simulink model "Neurofeedback_Full_fNIRS"  (R2021b)
settings: Solver=ode23tb  StartTime=0  StopTime=90  FixedStep=1/100  RelTol=1e-3
libraries: slpidlib x1
settings Model: Creator=mdls3  LastModifiedBy=mdls3
settings DataIOCC: SaveFormat=StructureWithTime
settings OptimizationCC: BlockReduction=off  BufferReuse=off
settings DebuggingCC: AlgebraicLoopMsg=none  UnconnectedInputMsg=none  UnconnectedOutputMsg=none  UnconnectedLineMsg=none  UnderSpecifiedDimensionMsg=warning

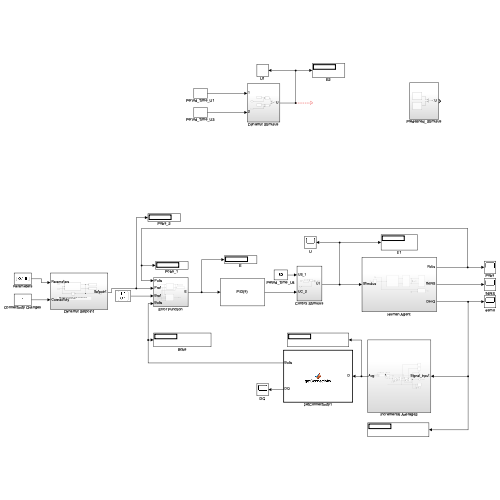
[thumbnail: Simulink's stored preview of the top-level diagram]
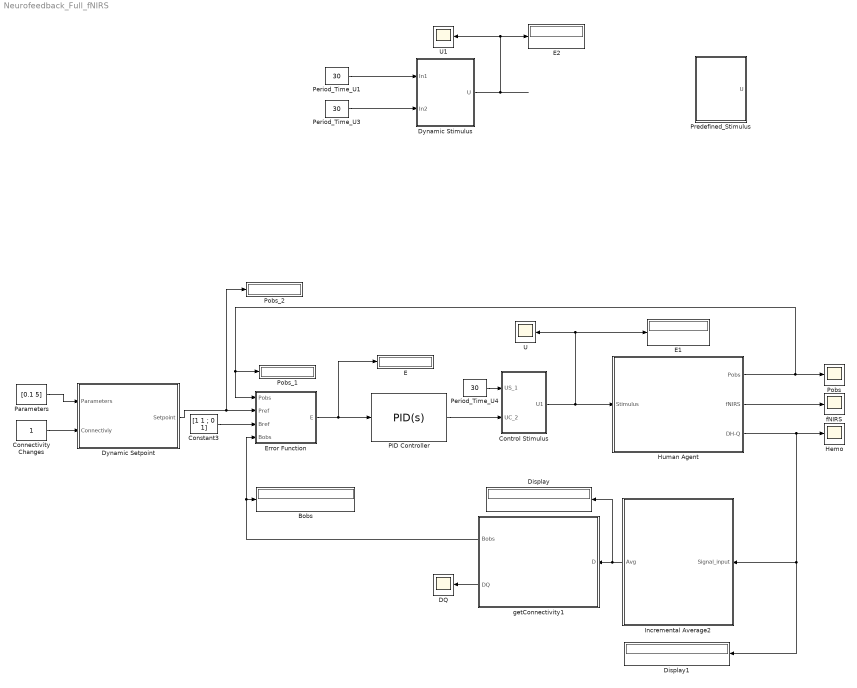
== system Neurofeedback_Full_fNIRS ==
  Bobs : Display
  Connectivity Changes : Constant
  Constant3 : Constant  Value="[1   1 ; 0  1]"
  Control Stimulus : Subsystem
  DQ : Scope
  Display : Display
  Display1 : Display
  Dynamic Setpoint : Subsystem
  Dynamic Stimulus : Subsystem
  E : Display
  E1 : Display
  E2 : Display
  Error Function : Subsystem
  Hemo : Scope
  Human Agent : Subsystem
  Incremental Average2 : Subsystem
  PID Controller : slpidlib/PID Controller  Controller=PID  Form=Ideal  TimeDomain=Continuous-time  UseExternalTs=off  SampleTime=-1  IntegratorMethod=Forward Euler  FilterMethod=Forward Euler  ControllerParametersSource=internal  P=0.3  I=0.12  D=0.85  UseFilter=on  N=100  TunerSelectOption=Transfer Function Based (PID Tuner App)  InitialConditionSource=internal  InitialConditionForIntegrator=0  InitialConditionForFilter=0  DifferentiatorICPrevScaledInput=0  ExternalReset=none  TrackingMode=off  Kt=1  LimitOutput=off  SatLimitsSource=internal  UpperSaturationLimit=inf  LowerSaturationLimit=-inf  LinearizeAsGain=on  AntiWindupMode=none  Kb=1  POutMin=[]  POutMax=[]  IOutMin=[]  IOutMax=[]  DOutMin=[]  DOutMax=[]  NOutMin=[]  NOutMax=[]  SumOutMin=[]  SumOutMax=[]  SaturationOutMin=[]  SaturationOutMax=[]  PParamMin=[]  PParamMax=[]  IParamMin=[]  IParamMax=[]  DParamMin=[]  DParamMax=[]  NParamMin=[]  NParamMax=[]  KbParamMin=[]  KbParamMax=[]  KtParamMin=[]  KtParamMax=[]  KbOutMin=[]  KbOutMax=[]  KtOutMin=[]  KtOutMax=[]  IntegratorOutMin=[]  IntegratorOutMax=[]  FilterOutMin=[]  FilterOutMax=[]  SumI1OutMin=[]  SumI1OutMax=[]  SumI2OutMin=[]  SumI2OutMax=[]  SumI3OutMin=[]  SumI3OutMax=[]  SumI4OutMin=[]  SumI4OutMax=[]  SumDOutMin=[]  SumDOutMax=[]  DifferentiatorOutMin=[]  DifferentiatorOutMax=[]  FilterDiffOutCoefMin=[]  FilterDiffOutCoefMax=[]  ReciprocalOutMin=[]  ReciprocalOutMax=[]  SumDenOutMin=[]  SumDenOutMax=[]  SumNumOutMin=[]  SumNumOutMax=[]  DivideOutMin=[]  DivideOutMax=[]  UdiffTsProdOutMin=[]  UdiffTsProdOutMax=[]  NTsProdOutMin=[]  NTsProdOutMax=[]  UintegralTsProdOutMin=[]  UintegralTsProdOutMax=[]  UngainTsProdOutMin=[]  UngainTsProdOutMax=[]  IntegratorContinuousStateAttributes=''  IntegratorStateMustResolveToSignalObject=off  IntegratorRTWStateStorageClass=Auto  FilterContinuousStateAttributes=''  FilterStateMustResolveToSignalObject=off  FilterRTWStateStorageClass=Auto  ParallelPVariant=Passthrough  IdealPVariant=InternalParameters  IVariant=InternalParameters  DVariant=InternalParameters  IntegratorVariant=Continuous  SatVariant=Disabled  AWVariant=Passthrough  PCopyVariant=Disabled  TRVariant=Disabled  FdbkBlocksVariant=Forward  IdealPFdbkVariant=Disabled  SatFdbkVariant=Disabled  DerivativeFilterVariant=ContFilter  NVariant=InternalParameters  NCopyVariant=Disabled  FilterICVariant=InternalICsFilter  IntegratorICVariant=InternalICs  ExternalResetVariant=Disabled  TRSumVariant=Passthrough  SumFdbkVariant=Disabled  SumVariant=Sum_PID  TsampFilterVariant=InternalTs  TsampNgainVariant=Passthrough  TsampIntegralVariant=Passthrough  ExternalSaturationOutDataTypeStr=Inherit: Same as second input
  Parameters : Constant  Value=[0.1 5]
  Period_Time_U1 : Constant  Value=30
  Period_Time_U3 : Constant  Value=30
  Period_Time_U4 : Constant  Value=30
  Pobs : Scope
  Pobs_1 : Display
  Pobs_2 : Display
  Predefined_Stimulus : Subsystem
  U : Scope
  U1 : Scope
  fNIRS : Scope
  getConnectivity1 : MATLAB Function  TreatAsAtomicUnit=on  SystemSampleTime=0
  wires:
  Constant3/1 -> Error Function/3(Bref)
  Dynamic Setpoint/1(Setpoint) -> Pobs_2/1, Error Function/2(Pref)
  Error Function/1(E) -> PID Controller/1, E/1
  Period_Time_U4/1 -> Control Stimulus/1(US_1)
  Period_Time_U1/1 -> Dynamic Stimulus/1(In1)
  Period_Time_U3/1 -> Dynamic Stimulus/2(In2)
  Dynamic Stimulus/1(U) -> E2/1, U1/1
  PID Controller/1 -> Control Stimulus/2(UC_2)
  Human Agent/1(Pobs) -> Pobs/1, Pobs_1/1, Error Function/1(Pobs)
  Human Agent/2(fNIRS) -> fNIRS/1
  Control Stimulus/1(U1) -> U/1, E1/1, Human Agent/1(Stimulus)
  Human Agent/3(DH-Q) -> Display1/1, Incremental Average2/1(Signal_input), Hemo/1
  Incremental Average2/1(Avg) -> Display/1, getConnectivity1/1("D ")
  getConnectivity1/2(DQ) -> DQ/1
  getConnectivity1/1(Bobs) -> Error Function/4(Bobs), Bobs/1
  Parameters/1 -> Dynamic Setpoint/1(Parameters)
  Connectivity Changes/1 -> Dynamic Setpoint/2(Connectiviy)

== system Neurofeedback_Full_fNIRS/Control Stimulus ==
  US_1 : Inport
  UC_2 : Inport  Port=2
  Duty_Cycle_U1 : Constant  Value=0.16667  OutMin=[0]  OutMax=[0.8]
  Mux : Mux  Inputs=2
  Variable Pulse Generator2 : VariablePulseGenerator  RunAtFixedTimeIntervals=on  SampleTime=1/100
  U1 : Outport
  wires:
  Duty_Cycle_U1/1 -> Variable Pulse Generator2/1
  US_1/1 -> Variable Pulse Generator2/2
  Variable Pulse Generator2/1 -> Mux/1
  UC_2/1 -> Mux/2
  Mux/1 -> U1/1

== system Neurofeedback_Full_fNIRS/Dynamic Setpoint ==
  note: It’s necessary to delete the random term and move it to change its connectivity changes.
  Parameters : Inport
  Connectiviy : Inport  Port=2
  Delay1 : Delay  DelayLength=1  InitialCondition=0
  MATLAB Function1 : MATLAB Function  TreatAsAtomicUnit=on
  Random : Display
  Set1 : Display
  Setpoint : Outport
  wires:
  Parameters/1 -> MATLAB Function1/1(Parameters)
  MATLAB Function1/2(random) -> Random/1
  MATLAB Function1/1(Setpoint) -> Set1/1, Setpoint/1, Delay1/1
  Delay1/1 -> MATLAB Function1/2(Last_pressure)
  Connectiviy/1 -> MATLAB Function1/3(Connectivity)

== system Neurofeedback_Full_fNIRS/Dynamic Stimulus ==
  In1 : Inport
  In2 : Inport  Port=2
  Duty_Cycle_U1 : Constant  Value=0.16667  OutMin=[0]  OutMax=[0.8]
  Duty_Cycle_U2 : Constant  Value=0.5  OutMin=[0]  OutMax=[0.8]
  Mux : Mux  Inputs=2
  Variable Pulse Generator1 : VariablePulseGenerator  RunAtFixedTimeIntervals=on  SampleTime=1/100
  Variable Pulse Generator2 : VariablePulseGenerator  RunAtFixedTimeIntervals=on  SampleTime=1/100
  U : Outport
  wires:
  In1/1 -> Variable Pulse Generator2/2
  Mux/1 -> U/1
  Variable Pulse Generator2/1 -> Mux/1
  Duty_Cycle_U1/1 -> Variable Pulse Generator2/1
  Duty_Cycle_U2/1 -> Variable Pulse Generator1/1
  In2/1 -> Variable Pulse Generator1/2
  Variable Pulse Generator1/1 -> Mux/2

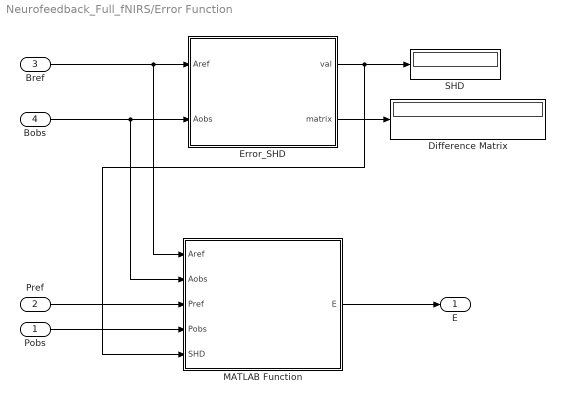
== system Neurofeedback_Full_fNIRS/Error Function ==
  Pobs : Inport
  Pref : Inport  Port=2
  Bref : Inport  Port=3
  Bobs : Inport  Port=4
  Difference Matrix : Display
  Error_SHD : MATLAB Function  TreatAsAtomicUnit=on
  MATLAB Function : MATLAB Function  TreatAsAtomicUnit=on
  SHD : Display
  E : Outport
  wires:
  Error_SHD/2(matrix) -> Difference Matrix/1
  Bref/1 -> MATLAB Function/1(Aref), Error_SHD/1(Aref)
  Error_SHD/1(val) -> SHD/1, MATLAB Function/5(SHD)
  MATLAB Function/1(E) -> E/1
  Bobs/1 -> MATLAB Function/2(Aobs), Error_SHD/2(Aobs)
  Pobs/1 -> MATLAB Function/4(Pobs)
  Pref/1 -> MATLAB Function/3(Pref)

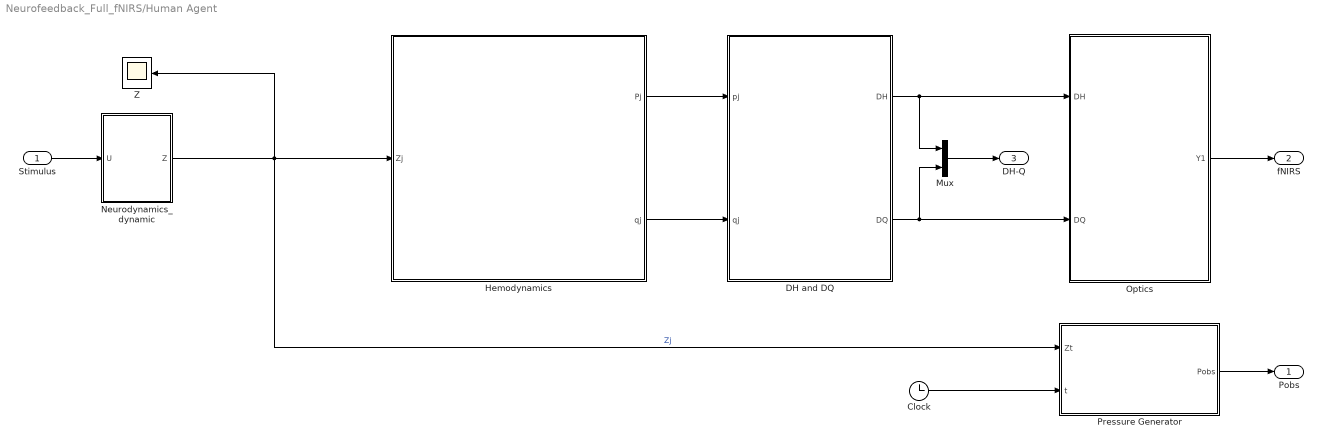
== system Neurofeedback_Full_fNIRS/Human Agent ==
  Stimulus : Inport
  Clock : Clock
  DH and DQ : Subsystem
  Hemodynamics : Subsystem
  Mux : Mux  Inputs=2
  Neurodynamics_dynamic : Subsystem
  Optics : Subsystem
  Pressure Generator : MATLAB Function  TreatAsAtomicUnit=on
  Z : Scope
  Pobs : Outport
  fNIRS : Outport  Port=2
  DH-Q : Outport  Port=3
  wires:
  Hemodynamics/1(Pj) -> DH and DQ/1(pj)
  Hemodynamics/2(qj) -> DH and DQ/2(qj)
  Neurodynamics_dynamic/1(Z) -> Hemodynamics/1(Zj), Z/1, Pressure Generator/1(Zt)  "Zj"
  DH and DQ/2(DQ) -> Mux/2, Optics/2(DQ)
  Optics/1(Y1) -> fNIRS/1
  Clock/1 -> Pressure Generator/2(t)
  Pressure Generator/1(Pobs) -> Pobs/1
  Stimulus/1 -> Neurodynamics_dynamic/1(U)
  DH and DQ/1(DH) -> Mux/1, Optics/1(DH)
  Mux/1 -> DH-Q/1

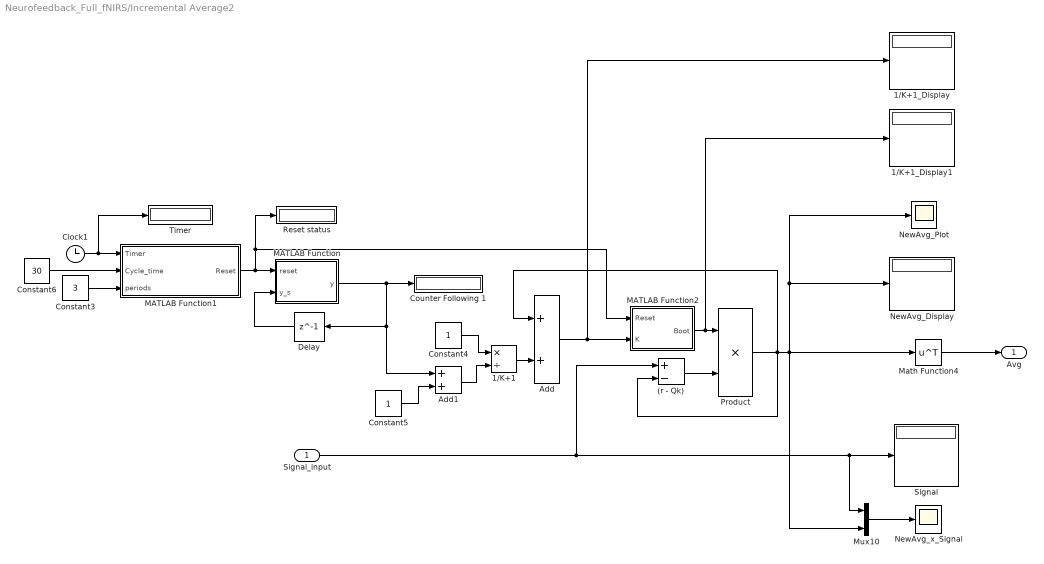
== system Neurofeedback_Full_fNIRS/Incremental Average2 ==
  Signal_input : Inport
  (r - Qk) : Sum  Inputs=+-
  1/K+1 : Product  Inputs=*/
  1/K+1_Display : Display
  1/K+1_Display1 : Display
  Add : Sum
  Add1 : Sum
  Clock1 : Clock
  Constant3 : Constant  Value=3
  Constant4 : Constant
  Constant5 : Constant
  Constant6 : Constant  Value=30
  Counter Following 1 : Display
  Delay : Delay  DelayLength=1  InitialCondition=0
  MATLAB Function : MATLAB Function  TreatAsAtomicUnit=on
  MATLAB Function1 : MATLAB Function  TreatAsAtomicUnit=on
  MATLAB Function2 : MATLAB Function  TreatAsAtomicUnit=on
  Math Function4 : Math  Operator=transpose  SaturateOnIntegerOverflow=on
  Mux10 : Mux  Inputs=2
  NewAvg_Display : Display
  NewAvg_Plot : Scope
  NewAvg_x_Signal : Scope
  Product : Product
  Reset status : Display
  Signal : Display
  Timer : Display
  Avg : Outport
  wires:
  (r - Qk)/1 -> Product/2
  Signal_input/1 -> Mux10/1, Signal/1, (r - Qk)/1
  Add/1 -> 1/K+1_Display/1, MATLAB Function2/2(K)
  Mux10/1 -> NewAvg_x_Signal/1
  Product/1 -> Add/1, (r - Qk)/2, Mux10/2, NewAvg_Plot/1, NewAvg_Display/1, Math Function4/1
  Math Function4/1 -> Avg/1
  Constant4/1 -> 1/K+1/1
  Constant5/1 -> Add1/2
  Add1/1 -> 1/K+1/2
  1/K+1/1 -> Add/2
  MATLAB Function/1(y) -> Delay/1, Add1/1, Counter Following 1/1
  Delay/1 -> MATLAB Function/2(y_s)
  MATLAB Function1/1(Reset) -> Reset status/1, MATLAB Function2/1(Reset), MATLAB Function/1(reset)
  Constant6/1 -> MATLAB Function1/2(Cycle_time)
  Constant3/1 -> MATLAB Function1/3(periods)
  Clock1/1 -> MATLAB Function1/1(Timer), Timer/1
  MATLAB Function2/1(Boot) -> 1/K+1_Display1/1, Product/1

== system Neurofeedback_Full_fNIRS/Predefined_Stimulus ==
  Mux : Mux  Inputs=2
  Pulse Generator : DiscretePulseGenerator  Amplitude=0.6  Period=30  PulseWidth=5
  Pulse Generator1 : DiscretePulseGenerator  Amplitude=0.6  Period=30  PulseWidth=6
  U : Outport
  wires:
  Mux/1 -> U/1
  Pulse Generator/1 -> Mux/1
  Pulse Generator1/1 -> Mux/2

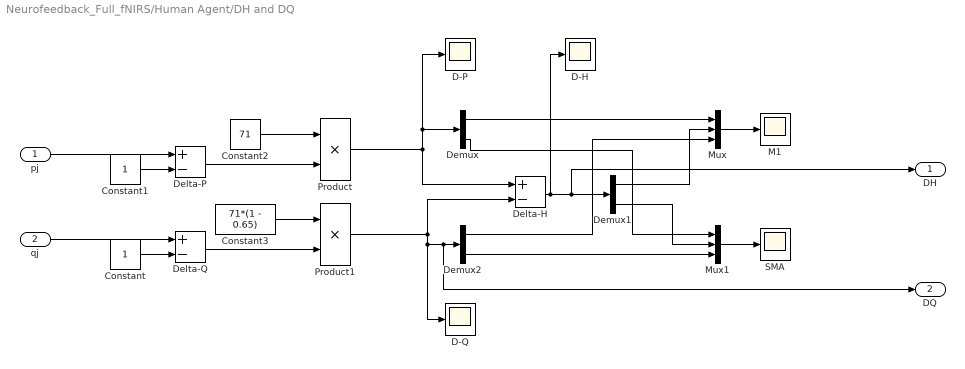
== system Neurofeedback_Full_fNIRS/Human Agent/DH and DQ ==
  pj : Inport
  qj : Inport  Port=2
  Constant : Constant
  Constant1 : Constant
  Constant2 : Constant  Value=71
  Constant3 : Constant  Value=71*(1 - 0.65)
  D-H : Scope
  D-P : Scope
  D-Q : Scope
  Delta-H : Sum  Inputs=+-
  Delta-P : Sum  Inputs=+-
  Delta-Q : Sum  Inputs=+-
  Demux : Demux  Outputs=2
  Demux1 : Demux  Outputs=2
  Demux2 : Demux  Outputs=2
  M1 : Scope
  Mux : Mux  Inputs=3
  Mux1 : Mux  Inputs=3
  Product : Product
  Product1 : Product
  SMA : Scope
  DH : Outport
  DQ : Outport  Port=2
  wires:
  Constant2/1 -> Product/1
  Delta-Q/1 -> Product1/2
  Constant3/1 -> Product1/1
  Demux2/2 -> Mux1/3
  pj/1 -> Delta-P/1
  Mux1/1 -> SMA/1
  Demux/2 -> Mux1/1
  Mux/1 -> M1/1
  Constant/1 -> Delta-Q/2
  Delta-P/1 -> Product/2
  Product1/1 -> DQ/1, Demux2/1, D-Q/1, Delta-H/2
  qj/1 -> Delta-Q/1
  Demux/1 -> Mux/1
  Delta-H/1 -> DH/1, Demux1/1, D-H/1
  Demux1/1 -> Mux/2
  Demux1/2 -> Mux1/2
  Product/1 -> Demux/1, D-P/1, Delta-H/1
  Demux2/1 -> Mux/3
  Constant1/1 -> Delta-P/2

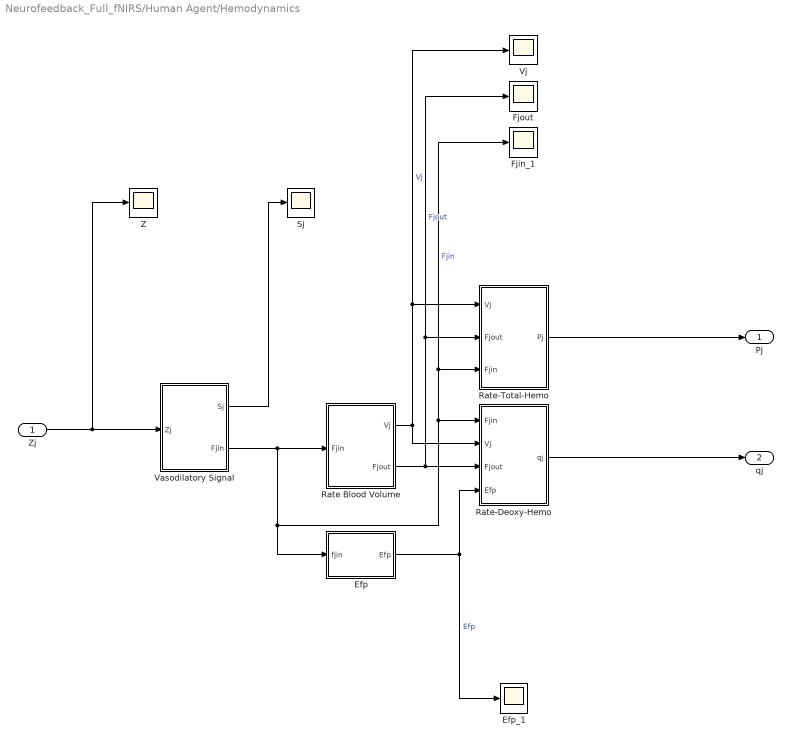
== system Neurofeedback_Full_fNIRS/Human Agent/Hemodynamics ==
  Zj : Inport
  Efp : MATLAB Function  TreatAsAtomicUnit=on
  Efp_1 : Scope
  Fjin_1 : Scope
  Fjout : Scope
  Rate Blood Volume : Subsystem
  Rate-Deoxy-Hemo : Subsystem
  Rate-Total-Hemo : Subsystem
  Sj : Scope
  Vasodilatory Signal : Subsystem
  Vj : Scope
  Z : Scope
  Pj : Outport
  qj : Outport  Port=2
  wires:
  Rate-Deoxy-Hemo/1(qj) -> qj/1
  Zj/1 -> Vasodilatory Signal/1(Zj), Z/1
  Vasodilatory Signal/1(Sj) -> Sj/1
  Rate Blood Volume/2(Fjout) -> Fjout/1, Rate-Total-Hemo/2(Fjout), Rate-Deoxy-Hemo/3(Fjout)  "Fjout"
  Rate Blood Volume/1(Vj) -> Vj/1, Rate-Total-Hemo/1(Vj), Rate-Deoxy-Hemo/2(Vj)  "Vj"
  Rate-Total-Hemo/1(Pj) -> Pj/1
  Efp/1(Efp) -> Rate-Deoxy-Hemo/4(Efp), Efp_1/1  "Efp"
  Vasodilatory Signal/2(Fjin) -> Efp/1(fjin), Fjin_1/1, Rate-Total-Hemo/3(Fjin), Rate-Deoxy-Hemo/1(Fjin), Rate Blood Volume/1(Fjin)  "Fjin"

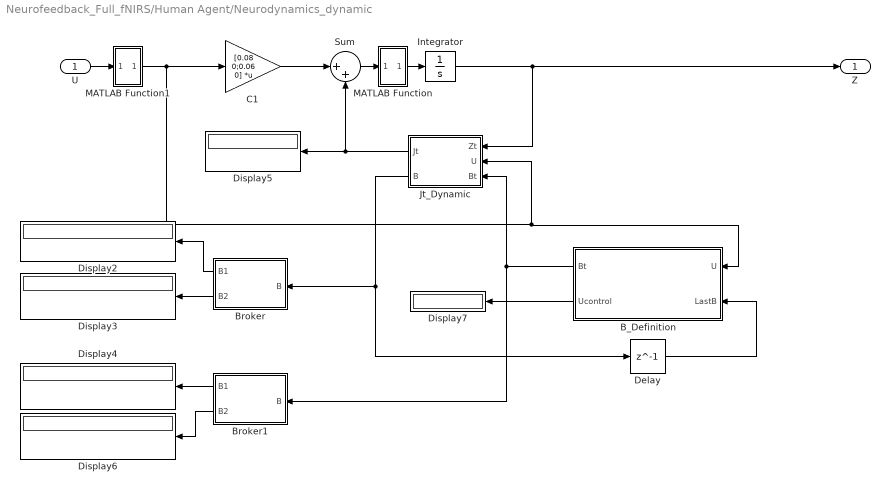
== system Neurofeedback_Full_fNIRS/Human Agent/Neurodynamics_dynamic ==
  U : Inport
  B_Definition : MATLAB Function  TreatAsAtomicUnit=on
  Broker : MATLAB Function  TreatAsAtomicUnit=on
  Broker1 : MATLAB Function  TreatAsAtomicUnit=on
  C1 : Gain  Gain=[0.08 0;0.06 0]  Multiplication=Matrix(K*u) (u vector)
  Delay : Delay  DelayLength=1  InitialCondition=0
  Display{2..7} (6 alike) : Display
  Integrator : Integrator
  Jt_Dynamic : MATLAB Function  TreatAsAtomicUnit=on
  MATLAB Function : MATLAB Function  TreatAsAtomicUnit=on
  MATLAB Function1 : MATLAB Function  TreatAsAtomicUnit=on
  Sum : Sum  Inputs=|++
  Z : Outport
  wires:
  Integrator/1 -> Z/1, Jt_Dynamic/1(Zt)
  C1/1 -> Sum/1
  U/1 -> MATLAB Function1/1(Z)
  Sum/1 -> MATLAB Function/1(Z)
  MATLAB Function1/1(Zn) -> C1/1, B_Definition/1(U), Jt_Dynamic/2(U)
  MATLAB Function/1(Zn) -> Integrator/1
  Jt_Dynamic/1(Jt) -> Display5/1, Sum/2
  Delay/1 -> B_Definition/2(LastB)
  Jt_Dynamic/2(B) -> Broker/1(B), Delay/1
  Broker/1(B1) -> Display2/1
  Broker/2(B2) -> Display3/1
  B_Definition/1(Bt) -> Broker1/1(B), Jt_Dynamic/3(Bt)
  Broker1/2(B2) -> Display6/1
  Broker1/1(B1) -> Display4/1
  B_Definition/2(Ucontrol) -> Display7/1

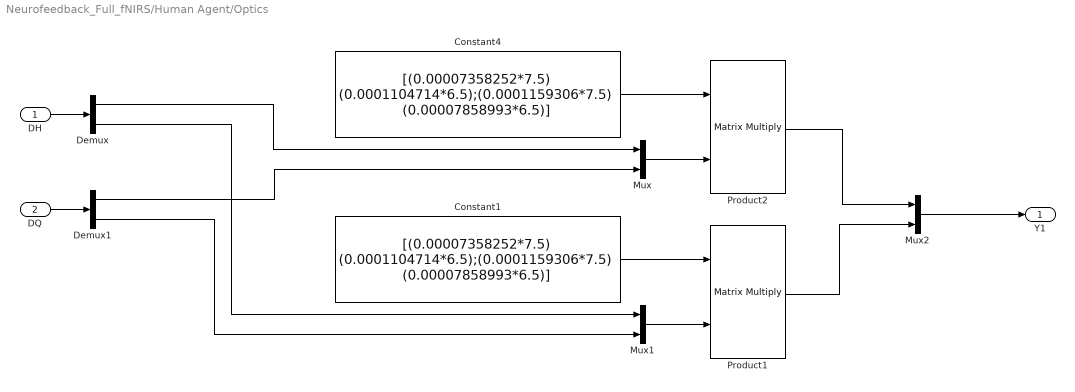
== system Neurofeedback_Full_fNIRS/Human Agent/Optics ==
  DH : Inport
  DQ : Inport  Port=2
  Constant1 : Constant  Value=[(0.00007358252*7.5) (0.0001104714*6.5);(0.0001159306*7.5) (0.00007858993*6.5)]
  Constant4 : Constant  Value=[(0.00007358252*7.5) (0.0001104714*6.5);(0.0001159306*7.5) (0.00007858993*6.5)]
  Demux : Demux  Outputs=2
  Demux1 : Demux  Outputs=2
  Mux : Mux  Inputs=2
  Mux1 : Mux  Inputs=2
  Mux2 : Mux  Inputs=2
  Product1 : Product  Multiplication=Matrix(*)
  Product2 : Product  Multiplication=Matrix(*)
  Y1 : Outport
  wires:
  Mux/1 -> Product2/2
  Product2/1 -> Mux2/1
  Mux1/1 -> Product1/2
  Product1/1 -> Mux2/2
  Constant1/1 -> Product1/1
  DH/1 -> Demux/1
  Demux/1 -> Mux/1
  Demux/2 -> Mux1/1
  DQ/1 -> Demux1/1
  Constant4/1 -> Product2/1
  Demux1/1 -> Mux/2
  Demux1/2 -> Mux1/2
  Mux2/1 -> Y1/1

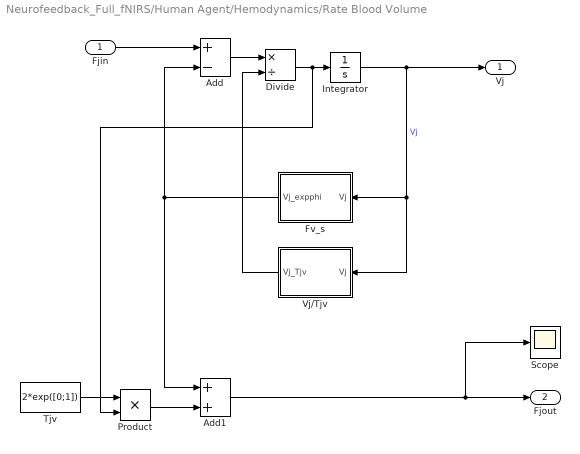
== system Neurofeedback_Full_fNIRS/Human Agent/Hemodynamics/Rate Blood Volume ==
  Fjin : Inport
  Add : Sum  Inputs=+-
  Add1 : Sum
  Divide : Product  Inputs=*/
  Fv_s : MATLAB Function  TreatAsAtomicUnit=on
  Integrator : Integrator  InitialCondition=exp([0;0])
  Product : Product
  Scope : Scope
  Tjv : Constant  Value=2*exp([0;1])
  Vj/Tjv : MATLAB Function  TreatAsAtomicUnit=on
  Vj : Outport
  Fjout : Outport  Port=2
  wires:
  Fjin/1 -> Add/1
  Integrator/1 -> Vj/1, Vj/Tjv/1(Vj), Fv_s/1(Vj)  "Vj"
  Divide/1 -> Product/2, Integrator/1
  Fv_s/1(Vj_expphi) -> Add/2, Add1/1
  Add/1 -> Divide/1
  Vj/Tjv/1(Vj_Tjv) -> Divide/2
  Product/1 -> Add1/2
  Tjv/1 -> Product/1
  Add1/1 -> Scope/1, Fjout/1

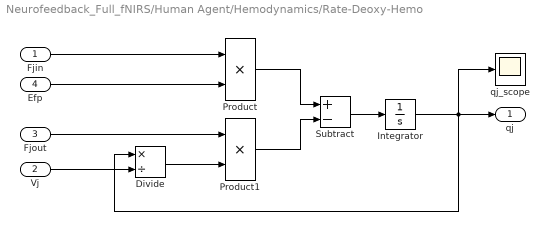
== system Neurofeedback_Full_fNIRS/Human Agent/Hemodynamics/Rate-Deoxy-Hemo ==
  Fjin : Inport
  Vj : Inport  Port=2
  Fjout : Inport  Port=3
  Efp : Inport  Port=4
  Divide : Product  Inputs=*/
  Integrator : Integrator  InitialCondition=exp([0;0])
  Product : Product
  Product1 : Product
  Subtract : Sum  Inputs=+-
  qj_scope : Scope
  qj : Outport
  wires:
  Efp/1 -> Product/2
  Divide/1 -> Product1/2
  Subtract/1 -> Integrator/1
  Integrator/1 -> qj/1, Divide/1, qj_scope/1
  Vj/1 -> Divide/2
  Product1/1 -> Subtract/2
  Fjin/1 -> Product/1
  Fjout/1 -> Product1/1
  Product/1 -> Subtract/1

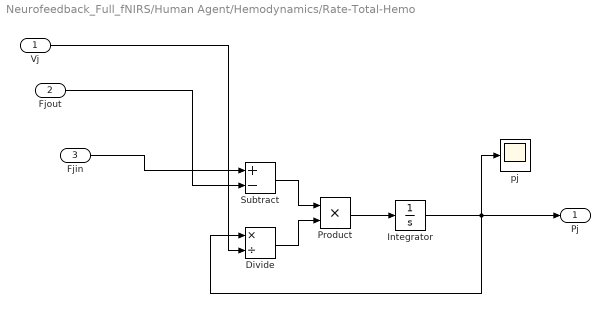
== system Neurofeedback_Full_fNIRS/Human Agent/Hemodynamics/Rate-Total-Hemo ==
  Vj : Inport
  Fjout : Inport  Port=2
  Fjin : Inport  Port=3
  Divide : Product  Inputs=*/
  Integrator : Integrator  InitialCondition=exp([0;0])
  Product : Product
  Subtract : Sum  Inputs=+-
  pj : Scope
  Pj : Outport
  wires:
  Fjout/1 -> Subtract/2
  Product/1 -> Integrator/1
  Vj/1 -> Divide/2
  Subtract/1 -> Product/1
  Fjin/1 -> Subtract/1
  Divide/1 -> Product/2
  Integrator/1 -> Pj/1, pj/1, Divide/1

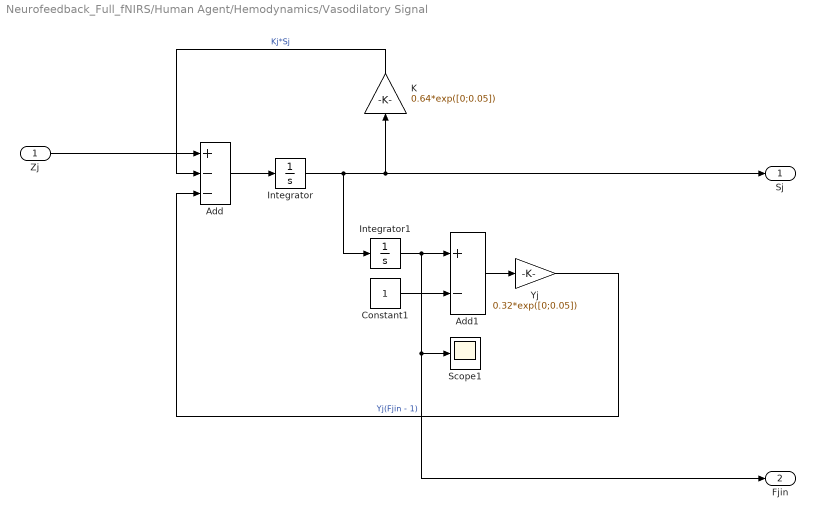
== system Neurofeedback_Full_fNIRS/Human Agent/Hemodynamics/Vasodilatory Signal ==
  Zj : Inport
  Add : Sum  Inputs=+--
  Add1 : Sum  Inputs=+-
  Constant1 : Constant
  Integrator : Integrator
  Integrator1 : Integrator  InitialCondition=exp([0;0])
  K : Gain  Gain=0.64*exp([0;0.05])
  Scope1 : Scope
  Yj : Gain  Gain=0.32*exp([0;0.05])
  Sj : Outport
  Fjin : Outport  Port=2
  wires:
  Add1/1 -> Yj/1
  K/1 -> Add/2  "Kj*Sj"
  Constant1/1 -> Add1/2
  Zj/1 -> Add/1
  Integrator1/1 -> Fjin/1, Scope1/1, Add1/1
  Integrator/1 -> Sj/1, K/1, Integrator1/1
  Add/1 -> Integrator/1
  Yj/1 -> Add/3  "Yj(Fjin - 1)"

== matlab function Neurofeedback_Full_fNIRS/Human Agent/Neurodynamics_dynamic/B_Definition ==
  settings: updateMethod=DISCRETE
  data: U input; Bt output; LastB input; Ucontrol output
function [Bt, Ucontrol] = B_Definition(U, LastB)
    Bt = zeros(2, 2, 2);
   %Control extraction and weight
   Ucontrol = U(2) * (0.2 + rand(1) * (1-0.2));
   Threshold = 0.2;
    if(Ucontrol < Threshold) %Random Ucontrol to test
        min = -1; 
        max = 1.5;
        n = 2;
        r1 = min + rand(n)*(max-min);
        r2 = min + rand(n)*(max-min);
        %Bt(:,:,1) = r1(:,:);
        Bt(:,:,2) = r2(:,:);
    else
       Bt = LastB;
    end

== matlab function Neurofeedback_Full_fNIRS/Human Agent/Neurodynamics_dynamic/Broker ==
  data: B input; B1 output; B2 output
function [B1, B2] = fcn(B)
B1 = B(:,:,1);
B2 = B(:,:,2);

== matlab function Neurofeedback_Full_fNIRS/Human Agent/Neurodynamics_dynamic/Broker1 ==
  data: B input; B1 output; B2 output
function [B1, B2] = fcn(B)
B1 = B(:,:,1);
B2 = B(:,:,2);

== matlab function Neurofeedback_Full_fNIRS/Human Agent/Neurodynamics_dynamic/Jt_Dynamic ==
  data: Zt input; U input; Jt output; Bt input; B output
function [Jt, B] = fcn(Zt, U, Bt)

   A = [-0.16 -0.49;-0.02 -0.33];
   nRegions  = size(A,1);

   B = zeros(2,2,2);
   a = 0;
   B1 = [0 0; 0 0]; %There must be a B per stimulus
   B2 = [-0.02 -0.77; 0.33 -1.31];

   if Bt(:,:,2) ~= B(:,:,2)
       B(:,:,:) = Bt(:,:,:);
   else
          B(:,:,1) = B1;
          B(:,:,2) = B2;
   end
   M = size(U,1); %nStimuli
   assert(M == size(B,3),...
        'Unexpected number of induced connectivity parameters B.');

    simulationLength = size(U,2);
    for t = 1:simulationLength
       T = zeros(nRegions); %nRegions x nRegions
                   for uu = 1:M % Sum (Uj * Bj)
                       tmp = U(uu,t) * B(:,:,uu);
                       T = -0.5 * exp(T + tmp);  
                   end
            SI = diag(A);
    end
        A =  A - diag(exp(SI) + (SI));
Jt = (A*Zt) + (T*Zt);

== matlab function Neurofeedback_Full_fNIRS/Incremental Average2/MATLAB Function ==
  data: reset input; y_s input; y output
function y = fcn(reset, y_s)

if reset == 1
    y = 0;
else 
    y = y_s + 1;
end

== matlab function Neurofeedback_Full_fNIRS/Human Agent/Neurodynamics_dynamic/MATLAB Function ==
  data: Z input; Zn output
function Zn = fcn(Z)

Zn = Z(:,1);

== matlab function Neurofeedback_Full_fNIRS/Human Agent/Neurodynamics_dynamic/MATLAB Function1 ==
  data: Z input; Zn output
function Zn = fcn(Z)

Zn = Z(:,1);

== matlab function Neurofeedback_Full_fNIRS/Incremental Average2/MATLAB Function1 ==
  data: Timer input; Reset output; Cycle_time input; periods input
function Reset  = fcn(Timer, Cycle_time, periods)

temp = 0;
PCycles = zeros(periods,1);
for i = 1:periods
    PCycles(i) = i * Cycle_time;
    if (Timer >= PCycles(i) && Timer <= PCycles(i)+1)
        temp = 1;
        break
    else
        temp = 0;
    end
end 
Reset = temp;

== matlab function Neurofeedback_Full_fNIRS/getConnectivity1 ==
  data: D input; Bobs output; DQ output
function [Bobs,DQ]  = getConnectivity(D)

    DQ = zeros(1, 2);
    DQ(1,1)=D(1,1);
    DQ(1,2)=D(1,2);


    DH = zeros(1,2);
    DH(1,1)=D(1,3);
    DH(1,2)=D(1,4);

    rThresh= 0.6; % [0..1] A threshold on the correlation.

    [nSamples, nChannels, nHb]=size(DQ);

    C = nan(nChannels, nChannels, nHb); %Matrix of channel pairwise correlations;

    %This part of the algorithm is HIGHLY inefficient but it does the job for now
    %but might not be sufficiently fast for "real time" neurofeedback

    for iHb = 1:nHb
        for iCh=1:nChannels
            for jCh=iCh:nChannels

                if iCh == jCh

                 C(iCh,jCh,iHb) = 1;

               else

                 C(iCh,jCh,iHb) = xcorr2(DQ(:,iCh,iHb),DQ(:,jCh,iHb));

                end
            end

        end

    end

    %Threshold/Binarize C


    tmp = C > rThresh;

    %Finally "merge" accross Hb species

    Bobs = all(tmp,3); %Apply the AND function across Hb species.

== matlab function Neurofeedback_Full_fNIRS/Error Function/Error_SHD ==
  data: Aref input; val output; Aobs input; matrix output
function [val,matrix]=SHD(Aref,Aobs)

val = sum(sum(xor(Aref,Aobs)));
matrix = xor(Aref,Aobs);

== matlab function Neurofeedback_Full_fNIRS/Human Agent/Hemodynamics/Efp ==
  data: fjin input; Efp output
function Efp= fcn(fjin)

Efp = (1 - (1 - 0.32).^ (1 ./ fjin))/0.32;

== matlab function Neurofeedback_Full_fNIRS/Error Function/MATLAB Function ==
  data: Aref input; E output; Aobs input; Pref input; Pobs input; SHD input
function E  = ErrorFunction(Aref, Aobs, Pref, Pobs, SHD)
    w1 = 0.1; %Use whatever values you like most. Threshold 

    w2 = 1 - w1;

    assert(all(size(Aref) == size(Aobs)));

    assert(size(Aref,1) == size(Aref,2));

    nChannels = size(Aref,1);

    AfullyConnected = ones(nChannels);

    AfullyDisconnected = zeros(nChannels);

    maxDiffSHD = sum(sum(xor(AfullyConnected,AfullyDisconnected))); %SHD

    errA = SHD/maxDiffSHD; %Normalize error in the connectivity

    errP = abs(Pobs-Pref)/abs(Pref);

    
E = w1 * errA + w2 * errP;

== matlab function Neurofeedback_Full_fNIRS/Human Agent/Hemodynamics/Rate Blood Volume/Fv_s ==
  data: Vj input; Vj_expphi output
function Vj_expphi = fcn(Vj)
phi = 0.32;
Vj_expphi = Vj.^(1/phi);

== matlab function Neurofeedback_Full_fNIRS/Human Agent/Hemodynamics/Rate Blood Volume/Vj//Tjv ==
  data: Vj input; Vj_Tjv output
function Vj_Tjv = fcn(Vj)
    Tjv = 2*exp([0;1]);
    Tj = 2*exp([0;0.05]);
Vj_Tjv =(Tj.*Tjv.*Vj);

== matlab function Neurofeedback_Full_fNIRS/Incremental Average2/MATLAB Function2 ==
  data: Reset input; K input; Boot output
function Boot = fcn(Reset, K)

    temp = ones(4, 1);
    Boot = [0;0;0;0];
    if Reset == 1
        temp = Boot;
    else 
        temp = K;
    end 

    Boot = temp;

== matlab function Neurofeedback_Full_fNIRS/Dynamic Setpoint/MATLAB Function1 ==
  settings: updateMethod=DISCRETE
  data: Setpoint output; Parameters input; Last_pressure input; random output; Connectivity input
function [Setpoint, random] = Random_Setpoint(Parameters, Last_pressure, Connectivity)
    %Parameters = [threshold Start_setpoint]
    temp = 0;
   %Pressure Setpoint selection
    pmin = 5;
    pmax = 8;
    new_pressure = pmin + rand(1)*(pmax-pmin);

    %Random used to simulate the connectivity changes, so we must change
    %the pressure setpoint when changes in the connectitvy are observed.
    min = 0;
    tmax = 10;
        %We should fine a random criteria to change the setpoint, not just
        %time, or the moment B changes. For now works to demostrate the
        %control without fNIRS
    random = min + rand(1) * (tmax - min) * new_pressure;
    if (Connectivity == 1)
         if (random < Parameters(1))
            %disp("Time")
            %disp(Time)
            temp = new_pressure;
            %disp("Setpoint")
            %disp(temp)
        else 
            temp = Last_pressure;
                if (Parameters(2) == temp || temp == 0)
                    temp = Parameters(2);
                else
                    temp = Last_pressure;
                end
         end  
    else
        temp = Parameters(2);
    end

    Setpoint = temp;

== matlab function Neurofeedback_Full_fNIRS/Human Agent/Pressure Generator ==
  data: Zt input; Pobs output; t input
function Pobs = fcn(Zt, t)
    R=28.2; %Resistor [Ohms];
    C=1.7; %Capacitor [Faradays];
    V= Zt(1); %Voltage or system reference;
    Vc = V * (exp(-t/(R*C))); % Voltage at the capacitor  
    
Pobs = Vc;
